simulink model "lattice"  (R2014b)
settings: Solver=ode45  StartTime=0.0  StopTime=10.0  RelTol=1e-3
settings Model: Creator=ravoson  LastModifiedBy=ravoson

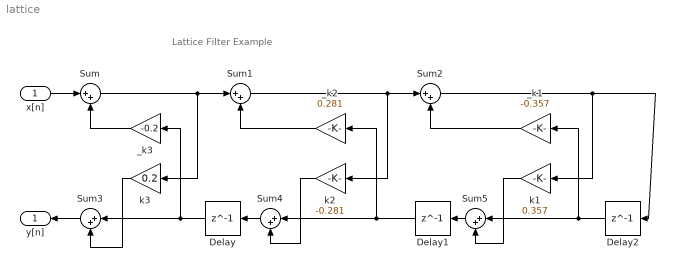
== system lattice ==
  note: Lattice Filter Example
  x[n] : Inport
  Delay : Delay  DelayLength=1  InitialCondition=0
  Delay1 : Delay  DelayLength=1  InitialCondition=0
  Delay2 : Delay  DelayLength=1  InitialCondition=0
  Sum{,1..5} (6 alike) : Sum  Inputs=|++
  _k1 : Gain  Gain=-0.357
  _k2 : Gain  Gain=0.281
  _k3 : Gain  Gain=-0.2
  k1 : Gain  Gain=0.357
  k2 : Gain  Gain=-0.281
  k3 : Gain  Gain=0.2
  y[n] : Outport
  wires:
  x[n]/1 -> Sum/1
  _k3/1 -> Sum/2
  Delay/1 -> Sum3/1, _k3/1
  Sum3/1 -> y[n]/1
  Sum/1 -> k3/1, Sum1/1
  Sum4/1 -> Delay/1
  _k2/1 -> Sum1/2
  Sum1/1 -> k2/1, Sum2/1
  Delay1/1 -> Sum4/1, _k2/1
  Sum5/1 -> Delay1/1
  _k1/1 -> Sum2/2
  Delay2/1 -> _k1/1, Sum5/1
  k1/1 -> Sum5/2
  k2/1 -> Sum4/2
  k3/1 -> Sum3/2
  Sum2/1 -> k1/1, Delay2/1
